simulink library "Mod_RLS"  (R2024b)
settings: Solver=VariableStepAuto  StartTime=0.0  StopTime=10.0  RelTol=1e-3
undefined symbols (not defined in the file or in its folder): Loop_V, P_V3, T
settings Model: Creator=Babaza_M  LastModifiedBy=Babaza_M

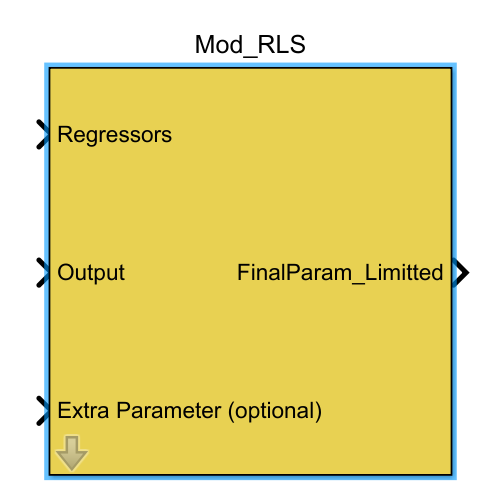
[thumbnail: Simulink's stored preview of the top-level diagram]
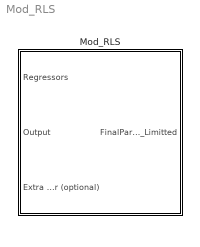
== system Mod_RLS ==
  Mod_RLS : Subsystem  Description=|  InitFcn=|  mask(Mod-RLS){nP=3, Init_V3=[-0.26  0.07 0.15], PPP=1e4, Pmax_coef=1, Pmin_coef=0.001, lambda_max=1, lambda_min=0.85, tau=1, T=T, H_Limits=[-1e-10 1000 1000], L_Limits=[-1000 1e-10 1e-10], RateActive=on, stopupdate_Value=off, Rate_Vec=[0.0002  0.0003 2], FinalParam0=[0.1 0.1 1000], H_R_Limits=[10 100 5000], L_R_Limits=[0 1e-6 1e-6]}
      Description=|
      | % Copyright (C) Dr. Mehrdad Babazadeh - WMG, University of Warwick, U.K. 10/12/2024 
      | % All Rights Reserved 
      | % This is the Betta version of Software that may be used with permission only
      InitFcn=|
      | ModelInitFcn
      | block_handle1 = find_system(bdroot, 'SearchDepth', Inf, 'Name',  'Mod_RLS'); 
      | block_handle = block_handle1{1}; 
      | 
      | %block_handles = find_system(bdroot, 'SearchDepth', Inf, 'BlockType', 'YourBlockType'); 
      | %if ~isempty(block_handles) block_handle = block_handles{1}; % Take the first found block % ... Your code using block_handle ... 
      | %else disp('Warning: Block of type "YourBlockType" not found.'); 
      | %end
      |    
      | nP = str2double (get_param(block_handle, 'nP')); 
      | Init_V3= eval (get_param(block_handle, 'Init_V3')); 
      | PPP = str2double (get_param(block_handle, 'PPP'));% 1e4 
      | Pmax_coef= str2double (get_param(block_handle, 'Pmax_coef'));% 1
      | Pmin_coef= str2double (get_param(block_handle, 'Pmin_coef'));% 0.75
      | 
      | lambda_min = eval (get_param(block_handle, 'lambda_min')); 
      | lambda_max = eval (get_param(block_handle, 'lambda_max')); 
      | tau = eval (get_param(block_handle, 'tau')); 
      | T = eval (get_param(block_handle, 'T')); 
      | 
      | RateActive= get_param(block_handle, 'RateActive'); 
      | Rate_Vec= eval (get_param(block_handle, 'Rate_Vec')); 
      | 
      | H_Limits = eval (get_param(block_handle, 'H_Limits')); 
      | L_Limits = eval (get_param(block_handle, 'L_Limits')); 
      | 
      | H_R_Limits = eval (get_param(block_handle, 'H_R_Limits')); 
      | L_R_Limits = eval (get_param(block_handle, 'L_R_Limits')); 
      | 
      | FinalParam0 = eval (get_param(block_handle, 'FinalParam0')); 
      | %FinalParam=FinalParam0;
      | %delta_Rate=FinalParam-FinalParam0;
      | %--------------------------------------------------------------------------------------
      | %% Inner Loops: 
      | Loop_V= 1; % 1; No of iteration of Inner loop (ECM) 
      |   
      | %% ECM: Initial values 
      | P_V3 = PPP * eye(nP);
      mask prompts: nP "Number of Parameters (n):"; Init_V3 "Initial Parameter Values:"; PPP "Parameter Covariance Matrix:"; Pmax_coef "Pmax coefficent:"; Pmin_coef "Pmin coefficent:"; T "Sample Time (only discrete):"; H_Limits "High limits intermediate params.:"; L_Limits "Low limits intermediate params.:"; RateActive "Rate Active:"; stopupdate_Value "stop update when input is zero"; Rate_Vec "Rate Vector:"; FinalParam0 "Initial values of Final params.:"; H_R_Limits "High limits Final params.:"; L_R_Limits "Low limits Final params.:"
      mask help:
      | Description:
      | This masked block implements a Modified Recursive Least Square (Mod_RLS) technique for real-time parameter identification of either linear or nonlinear system identification.
      |
      | Important notice (Naming standard):
      |     If there is only one Mod_RLS block, it's name has to be unchanged.
      |     If there are several similar blocks, one of them has to be named 'Mod_RLS'. The others can be Mod_RLSX where X can be whatever name.
      mask Help:
      | Description:
      | This masked block implements a Modified Recursive Least Square (Mod_RLS) technique for real-time parameter identification of either linear or nonlinear system identification.
      | Considering a regression equation structure, this block takes a vector of regressors, an output, and a few initial settings. Thereafter, unknown ‘intermediate parameters’ are calculated based on a modified recursive least square with adaptive forgetting factor.
      | 
      | Important notice:
      | Naming standard:
      |     If there is only one Mod_RLS block, it's name has to be unchanged.
      |     If there are several similar blocks, one of them has to be named 'Mod_RLS'. The others can be Mod_RLSX where X can be whatever name.
      | 
      | There are two types of unknown parameters in this method:
      | 1. A vector of independent, intermediate parameters such as: alpha, betta, gamma, ...
      | 2. A vector of dependent, final parameters such as R0. R1, C1, ... that are dependent on intermediate parameters. For example:
      | R0 = f(alpha, beta, gamma,…)
      | R1= g((alpha, beta, gamma,…)
      | …
      | 
      | Important Characteristics of Mod_RLS:
      | 1. Since, this method might be used for nonlinear system identification, setting some limits are available to help preventing local minimums.
      | 2. ‘Final parameters’ are dependent on the ‘intermediate parameters’ that can be defined appropriately in an internal block named ‘User defined Relations'. An example of this in the following:
      | 
      | function FinalParam   = fcn(Theta_New, FinalParam, ExtraParam)
      |     meu= Theta_New(2)/(Theta_New(1)*ExtraParam);
      |     FinalParam(1)= -Theta_New(1)*meu^2/(Theta_New(2)*(Theta_New(3)*meu+Theta_New(2)));
      |     FinalParam(2)= -Theta_New(1)/Theta_New(2);
      |     FinalParam(3)= -(Theta_New(3)+Theta_New(2)/meu)/Theta_New(1);
      | 
      | Settings:
      | Number of Parameters (n): Number of unknown parameters
      | Initial Parameter Values
      | P(0): Initial error covariance matrix coefficient. For exam if n=2 and P(0)= 1e4 means P=[1e4 0 ; 0 1e4].
      | Pmax coefficient: To determine maximum value of covariance matrix P to reset to the initial value.
      | Pmin coefficient: To determine minimum value of covariance matrix P to reset to the initial value.
      | lambda_min, lambda_max, and tau are values to set adaptive forgetting factor method.
      | Relation for adaptive forgetting factor is:
      | Lambda = lambda_min + (lambda_max - lambda_min) * exp(-tau * abs(error));
      | 
      | Sample Time (only discrete): This value determines the sampling time of the block
      | High limits intermediate params.: To freeze higher band of intermediate parameters
      | Low limits intermediate params.: To freeze lower band of intermediate parameters
      | Rate Active: To activate or deactivate rate limits on Final parameters
      | Rate Vector: To set the allowed absolute rate of change in Final parameters
      | Initial values of Final params.: To determine starting point in rate limits
      | High limits Final params
      | Low limits Final params
      | 
      | Inputs:
      | Vector of Regressors
      | Output of regression equation
      | Extra parameter (optional): This might be a constant or variable parameter or a vector of parameters to be used in ‘User defined Relations' for extra flexibility.
      | 
      | Instruction:
      | Connect the Inputs to the input ports of the block.
      | Adjust the values and limits to tune the Mod_RLS response.
      | Connect the output port to the relevant scope.
      | Define the relationship between ‘Final parameters’ and ‘Intermediate Parameters’.
      mask DialogControl Container2 Prompt: Initial values
      mask DialogControl Init_V3 Tooltip: Initial parameters for discrete-time unknown intermediate parameters
      mask DialogControl PPP Tooltip: Scalar coefficient
      mask DialogControl Pmax_coef Tooltip: After this point is approached by P, it will be reset to initial value
      mask DialogControl Pmin_coef Tooltip: After this point is approached by P, it will be reset to initial value
      mask DialogControl lambda_max Tooltip: To be used in Adaptive forgetting factor
      mask DialogControl lambda_min Tooltip: To be used in Adaptive forgetting factor
      mask DialogControl tau Tooltip: To be used in Adaptive forgetting factor
      mask DialogControl Container4 Prompt: Freezing Limits on intermediate params.
      mask DialogControl H_Limits Tooltip: If either of parameters approach these values, the previous appropriate value will be effective
      mask DialogControl L_Limits Tooltip: If either of parameters approach these values, the previous appropriate value will be effective
      mask DialogControl Container5 Prompt: Limits on Final params.
      mask DialogControl RateActive Tooltip: To activate/deactivate rate on the Final parameters
      mask DialogControl FinalParam0 Tooltip: Starting point of Final parameters
      mask DialogControl H_R_Limits Tooltip: Maximum value for Final parameters to show
      mask DialogControl L_R_Limits Tooltip: Minimum value for Final parameters to show

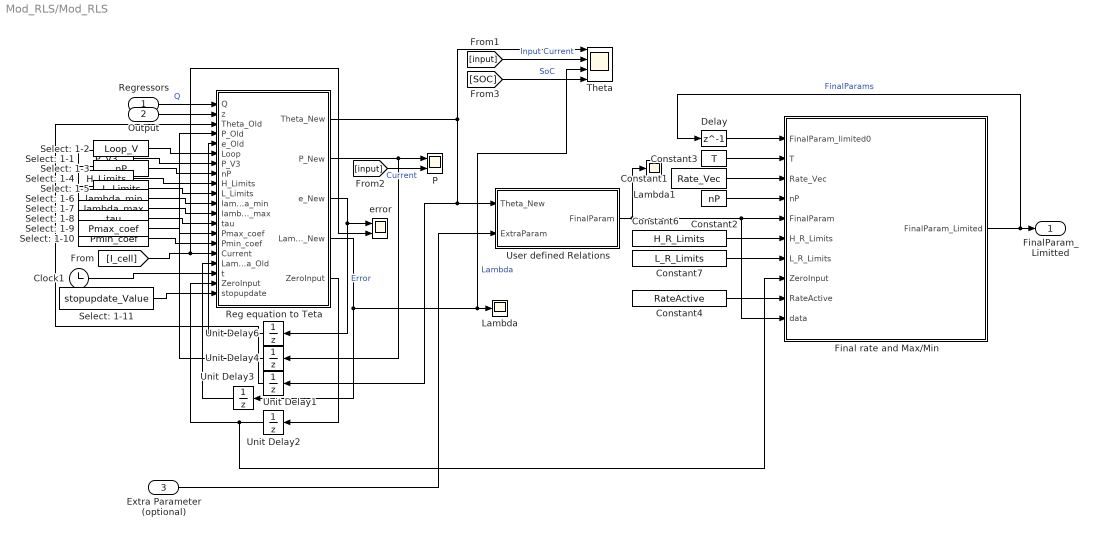
== system Mod_RLS/Mod_RLS ==
  Regressors : Inport
  Output : Inport  Port=2
  Extra Parameter (optional) : Inport  Port=3
  Clock1 : Clock
  Constant1 : Constant  Value=Rate_Vec  SampleTime=T
  Constant2 : Constant  Value=nP  SampleTime=T
  Constant3 : Constant  Value=T  SampleTime=T
  Constant4 : Constant  Value=RateActive  SampleTime=T
  Constant6 : Constant  Value=H_R_Limits  SampleTime=T
  Constant7 : Constant  Value=L_R_Limits  SampleTime=T
  Delay : Delay  DelayLength=1  InitialCondition=FinalParam0  SampleTime=T
  Final rate and Max/Min : MATLAB Function  TreatAsAtomicUnit=on
  Lambda : Scope
  Lambda1 : Scope
  P : Scope  NumInputPorts=2
  Reg equation to Teta : MATLAB Function  TreatAsAtomicUnit=on  SystemSampleTime=T
  Select: 1-1 : Constant  Value=P_V3  SampleTime=T
  Select: 1-10 : Constant  Value=Pmin_coef  SampleTime=T
  Select: 1-11 : Constant  Value=stopupdate_Value  SampleTime=T
  Select: 1-2 : Constant  Value=Loop_V  SampleTime=T
  Select: 1-3 : Constant  Value=nP  SampleTime=T
  Select: 1-4 : Constant  Value=H_Limits  SampleTime=T
  Select: 1-5 : Constant  Value=L_Limits  SampleTime=T
  Select: 1-6 : Constant  Value=lambda_min  SampleTime=T
  Select: 1-7 : Constant  Value=lambda_max  SampleTime=T
  Select: 1-8 : Constant  Value=tau  SampleTime=T
  Select: 1-9 : Constant  Value=Pmax_coef  SampleTime=T
  Theta : Scope  NumInputPorts=4
  Unit Delay1 : UnitDelay  InitialCondition=Init_V3  SampleTime=T  HasFrameUpgradeWarning=on
  Unit Delay2 : UnitDelay  InitialCondition=stopupdate_Value  SampleTime=T  HasFrameUpgradeWarning=on
  Unit Delay3 : UnitDelay  InitialCondition=1  SampleTime=T  HasFrameUpgradeWarning=on
  Unit Delay4 : UnitDelay  InitialCondition=P_V3  SampleTime=T  HasFrameUpgradeWarning=on
  Unit Delay6 : UnitDelay  SampleTime=T  HasFrameUpgradeWarning=on
  User defined Relations : MATLAB Function  TreatAsAtomicUnit=on
  error : Scope  NumInputPorts=2
  FinalParam_Limitted : Outport
  wires:
  Constant1/1 -> Final rate and Max/Min/3(Rate_Vec)
  [SOC] -> Theta/4  "SoC"
  [input] -> P/2  "Current"
  Clock1/1 -> Reg equation to Teta/18(t)
  [input] -> Theta/2  "Input Current"
  Delay/1 -> Final rate and Max/Min/1(FinalParam_limited0)
  [I_cell] -> Reg equation to Teta/16(Current), error/2
  Unit Delay3/1 -> Reg equation to Teta/17(Lambda_Old)
  Extra Parameter (optional)/1 -> User defined Relations/2(ExtraParam)
  Select: 1-10/1 -> Reg equation to Teta/15(Pmin_coef)
  Select: 1-9/1 -> Reg equation to Teta/14(Pmax_coef)
  User defined Relations/1(FinalParam) -> Lambda1/1, Final rate and Max/Min/5(FinalParam), Final rate and Max/Min/10(data)
  Constant7/1 -> Final rate and Max/Min/7(L_R_Limits)
  Constant6/1 -> Final rate and Max/Min/6(H_R_Limits)
  Constant2/1 -> Final rate and Max/Min/4(nP)
  Select: 1-8/1 -> Reg equation to Teta/13(tau)
  Select: 1-7/1 -> Reg equation to Teta/12(lambda_max)
  Select: 1-6/1 -> Reg equation to Teta/11(lambda_min)
  Select: 1-5/1 -> Reg equation to Teta/10(L_Limits)
  Select: 1-4/1 -> Reg equation to Teta/9(H_Limits)
  Select: 1-3/1 -> Reg equation to Teta/8(nP)
  Reg equation to Teta/4(Lambda_New) -> Unit Delay3/1, Lambda/1, Theta/3  "Lambda"
  Reg equation to Teta/2(P_New) -> P/1, Unit Delay4/1
  Final rate and Max/Min/1(FinalParam_Limited) -> Delay/1, FinalParam_Limitted/1  "FinalParams"
  Reg equation to Teta/1(Theta_New) -> User defined Relations/1(Theta_New), Unit Delay1/1, Theta/1
  Unit Delay6/1 -> Reg equation to Teta/5(e_Old)
  Unit Delay1/1 -> Reg equation to Teta/3(Theta_Old)
  Select: 1-2/1 -> Reg equation to Teta/6(Loop)
  Select: 1-1/1 -> Reg equation to Teta/7(P_V3)
  Unit Delay4/1 -> Reg equation to Teta/4(P_Old)
  Reg equation to Teta/3(e_New) -> error/1, Unit Delay6/1  "Error"
  Constant3/1 -> Final rate and Max/Min/2(T)
  Output/1 -> Reg equation to Teta/2(z)
  Regressors/1 -> Reg equation to Teta/1(Q)  "Q"
  Reg equation to Teta/5(ZeroInput) -> Unit Delay2/1
  Unit Delay2/1 -> Final rate and Max/Min/8(ZeroInput), Reg equation to Teta/19("ZeroInput ")
  Select: 1-11/1 -> Reg equation to Teta/20(stopupdate)
  Constant4/1 -> Final rate and Max/Min/9(RateActive)

== matlab function Mod_RLS/Reg equation to Teta ==
  data: Q input; z input; Theta_Old input; Theta_New output; P_Old input; e_Old input; P_New output; e_New output; Loop input; P_V3 input; Lambda_New output; nP input; H_Limits input; L_Limits input; lambda_min input; lambda_max input; tau input; Pmax_coef input; Pmin_coef input; Current input; Lambda_Old input; t input; ZeroInput output; ZeroInput input; stopupdate input
function [Theta_New, P_New, e_New, Lambda_New, ZeroInput]  = fcn(Q, z, Theta_Old, P_Old, e_Old, Loop, P_V3, nP, H_Limits, L_Limits,lambda_min, lambda_max, tau, Pmax_coef, Pmin_coef, Current,Lambda_Old, t,ZeroInput,stopupdate)
     
    ThetaM = Theta_Old;
    Theta_New= Theta_Old;
    Lambda_New = Lambda_Old;
    % if (t>961 || t<=962)
    %     ss=0;
    % end
    % The following lines guarantyies two cases with/without stop updateduring input =0
    if (stopupdate==1)
        if (abs(Current) > 0.001)
            ZeroInput=0;
        else
           ZeroInput=1;
        % elseif (abs(Current) ==0)
        %     ZeroInput=1;        
        end
    else
        ZeroInput=0;
    end

    if (ZeroInput==1)
        P_New = P_Old;
        e_New = e_Old;
        Lambda_New = Lambda_Old;        
    else

        e_New = e_Old;        
        P_New = P_Old;        
        %z_hat= 0;
    
        %%
        C= Pmax_coef*P_V3 (1,1);
        B= Pmin_coef*P_V3 (1,1);
        
        for i=1:nP
            if (abs(P_New(i,i)) < B || abs(P_New(i,i)) > C)
                P_New= P_V3;
                break; 
            end
        end 
    
        %% Algorithm 4        
        I1 = eye(nP);
        % tau= 1; % To test locally
    
        for i=1:Loop                
            z_hat = Q' * Theta_Old;
            e_New = z - z_hat;
            % Calculate gain with variable forgetting factor
            Lambda_New = lambda_min + (lambda_max - lambda_min) * exp(-tau * abs(e_New));
            
            K = P_New * Q * (Lambda_New + Q' * P_New * Q)^-1;
            Theta_New = Theta_Old + K * e_New;
            P_New = (I1 - K * Q') * P_New / Lambda_New;
        end
    
        %% Apply Freezing limits on intermediate parameters
            
        % The following values causes alpha, beta, and gamma don't change to critical values    
        % this condition is better than limiting values because different
        % parameters may need different limits
        
        for i=1:nP
            if (Theta_New(i)>= H_Limits(i) || Theta_New(i)<= L_Limits(i))   
                Theta_New= ThetaM;
                break;
            end
        end
    end

== matlab function Mod_RLS/User defined Relations ==
  data: FinalParam output; Theta_New input; ExtraParam input
function FinalParam   = fcn(Theta_New, ExtraParam)

FinalParam = zeros(1, 3); % Or zeros(3, 1) for a column vector
FinalParam(1)= Theta_New(3);
FinalParam(2)= -(Theta_New(3)+Theta_New(2)/Theta_New(1));  
FinalParam(3)= 1/(Theta_New(2)+Theta_New(1)*Theta_New(3));

== matlab function Mod_RLS/Final rate and Max//Min ==
  data: FinalParam_limited0 input; FinalParam_Limited output; T input; Rate_Vec input; nP input; FinalParam input; H_R_Limits input; L_R_Limits input; ZeroInput input; RateActive input; data input
function FinalParam_Limited  = fcn(FinalParam_limited0, T, Rate_Vec, nP, FinalParam, H_R_Limits, L_R_Limits, ZeroInput, RateActive, data)
% Bringing FinalParam is needed. Othervise we get error

%%  Calculation

delta_Rate = (FinalParam -FinalParam_limited0)/T;
FinalParam_Limited = FinalParam_limited0;  % Negative rate limit

%% Rate and Max/Min Limits
if (ZeroInput==1)
    FinalParam_Limited=FinalParam_limited0;
else
    for i=1:nP
        delta_Rate(i) = (FinalParam(i) - FinalParam_limited0(i))/T;
        if (RateActive==1)
            if delta_Rate(i) > Rate_Vec(i) 
                FinalParam_Limited(i) = FinalParam_limited0(i) + Rate_Vec(i)*T ;  % Positive rate limit
            elseif (delta_Rate(i) >=0 &&  delta_Rate(i) <= Rate_Vec(i)) 
                FinalParam_Limited(i) = FinalParam_limited0(i) + delta_Rate(i)*T ;  % Positive rate limit
            
            elseif delta_Rate(i) < -Rate_Vec(i) 
                FinalParam_Limited(i) = FinalParam_limited0(i) - Rate_Vec(i)*T;  % Negative rate limit
            elseif (delta_Rate(i) <0 &&  delta_Rate(i) >= -Rate_Vec(i)) 
                FinalParam_Limited(i) = FinalParam_limited0(i) + delta_Rate(i)*T ;  % Positive rate limit

            end
        else
            FinalParam_Limited(i)=FinalParam(i);            
        end

        if FinalParam_Limited(i) > H_R_Limits(i)
            FinalParam_Limited(i)= H_R_Limits(i);
        end
        if FinalParam_Limited(i)<L_R_Limits(i)
            FinalParam_Limited(i)= L_R_Limits(i);
        end
    end
end
